simulink model "FullSystemSimFinal_sexy"  (R2020a)
settings: Solver=ode23t  StartTime=0.0  StopTime=T_sim  MaxStep=0.0005  RelTol=1e-3
values from neighbouring files (symbols this model uses):
  a_friction = 0    [FullSystem.m]
  b_friction = 1.19    [FullSystem.m]
  C_T_matrix = ex2(2:12,2:12)'    [FullSystem.m]
  d_turbine = 0.15    [FullSystem.m]
  I_mp_data = ex4(:,5)    [FullSystem.m]
  I_sc_data = ex4(:,3)    [FullSystem.m]
  J_wind = 5.245e-6 * 1000    (= 0.005245)    [FullSystem.m]
  K_t = 0.023    [FullSystem.m]    (also in WindTurbine.m = 82.8991502528)
  K_v = 0.023 * pi / 30    (= 0.00240855436775)    [FullSystem.m]    (also in WindTurbine.m = 115.191730632)
  lambda_data_x = ex3(3, :)'    [FullSystem.m]
  lambda_opt = 2.8    [FullSystem.m]
  omega_0 = 1000    [FullSystem.m]    (also in SystemControl_script.m = 100:)
  P_max_EL = 3    [FullSystem.m]
  P_max_FC = 1    [FullSystem.m]
  R_LED_max = 75/4    (= 18.75)    [FullSystem.m]
  r_LED_x = ex1(4, :)'    [FullSystem.m]
  R_mp_data = ex4(:,6)    [FullSystem.m]
  r_PS_x = ex1(5,:)'    [FullSystem.m]
  r_solar_data_x = ex4(:,1)    [FullSystem.m]
  r_SP_x = ex1(3, :)'    [FullSystem.m]
  r_wind_data_x = ex3(1, :)'    [FullSystem.m]
  r_WT_x = ex1(2, :)'    [FullSystem.m]
  rho_air = 1.225    [FullSystem.m]
  step_size = T_sim/n    (= 0.01)    [FullSystem.m]
  T_sim = 10    [FullSystem.m]    (also in SystemControl_script.m; model_1.m = 24)
  V_mp_data = ex4(:,4)    [FullSystem.m]
  V_oc_data = ex4(:,2)    [FullSystem.m]
  V_w_data_x = ex3(2,:)'    [FullSystem.m]
undefined symbols (not defined in the file or in its folder): DiscIntNeverNeededParam
libraries: fl_lib x54, nesl_utility x49, simulink x2, ee_lib x1
settings Model: Creator=thequ  LastModifiedBy=thequ
settings DebuggingCC: SignalInfNanChecking=warning  ArithmeticOperatorsInVariantConditions=warning
settings SFSimCC: CustomCodeUndefinedFunction=UseInterfaceOnly

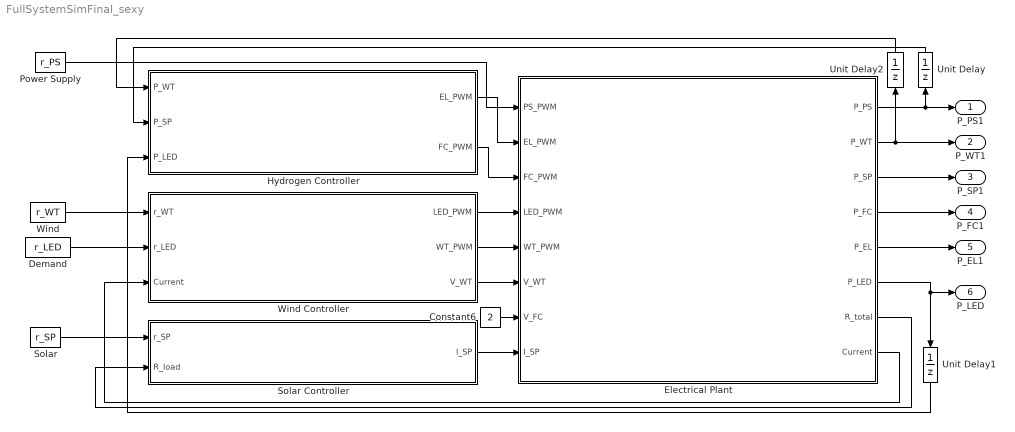
== system FullSystemSimFinal_sexy ==
  Constant6 : Constant  Value=2
  Demand : FromWorkspace  VariableName=r_LED  SampleTime=T_sim/length(r_LED_x)  Interpolate=off  OutputAfterFinalValue=Holding final value
  Electrical Plant : Subsystem
  Hydrogen Controller : Subsystem
  Power Supply : FromWorkspace  VariableName=r_PS  SampleTime=T_sim/length(r_PS_x)  Interpolate=off  OutputAfterFinalValue=Holding final value
  Solar : FromWorkspace  VariableName=r_SP  SampleTime=T_sim/length(r_SP_x)  Interpolate=off  OutputAfterFinalValue=Holding final value
  Solar Controller : Subsystem
  Unit Delay : UnitDelay  SampleTime=-1  HasFrameUpgradeWarning=on
  Unit Delay1 : UnitDelay  SampleTime=-1  HasFrameUpgradeWarning=on
  Unit Delay2 : UnitDelay  SampleTime=-1  HasFrameUpgradeWarning=on
  Wind : FromWorkspace  VariableName=r_WT  SampleTime=T_sim/length(r_WT_x)  Interpolate=off  OutputAfterFinalValue=Holding final value
  Wind Controller : Subsystem
  P_PS1 : Outport
  P_WT1 : Outport  Port=2
  P_SP1 : Outport  Port=3
  P_FC1 : Outport  Port=4
  P_EL1 : Outport  Port=5
  P_LED : Outport  Port=6
  wires:
  Electrical Plant/1(P_PS) -> P_PS1/1, Unit Delay/1
  Electrical Plant/2(P_WT) -> P_WT1/1, Unit Delay2/1
  Electrical Plant/3(P_SP) -> P_SP1/1
  Electrical Plant/4(P_FC) -> P_FC1/1
  Electrical Plant/5(P_EL) -> P_EL1/1
  Demand/1 -> Wind Controller/2(r_LED)
  Constant6/1 -> Electrical Plant/7(V_FC)
  Wind/1 -> Wind Controller/1(r_WT)
  Wind Controller/2(WT_PWM) -> Electrical Plant/5(WT_PWM)
  Power Supply/1 -> Electrical Plant/1(PS_PWM)
  Hydrogen Controller/1(EL_PWM) -> Electrical Plant/2(EL_PWM)
  Hydrogen Controller/2(FC_PWM) -> Electrical Plant/3(FC_PWM)
  Wind Controller/1(LED_PWM) -> Electrical Plant/4(LED_PWM)
  Wind Controller/3(V_WT) -> Electrical Plant/6(V_WT)
  Electrical Plant/8(Current) -> Wind Controller/3(Current)
  Electrical Plant/6(P_LED) -> P_LED/1, Unit Delay1/1
  Unit Delay/1 -> Hydrogen Controller/2(P_SP)
  Unit Delay1/1 -> Hydrogen Controller/3(P_LED)
  Unit Delay2/1 -> Hydrogen Controller/1(P_WT)
  Solar Controller/1(I_SP) -> Electrical Plant/8(I_SP)
  Solar/1 -> Solar Controller/1(r_SP)
  Electrical Plant/7(R_total) -> Solar Controller/2(R_load)

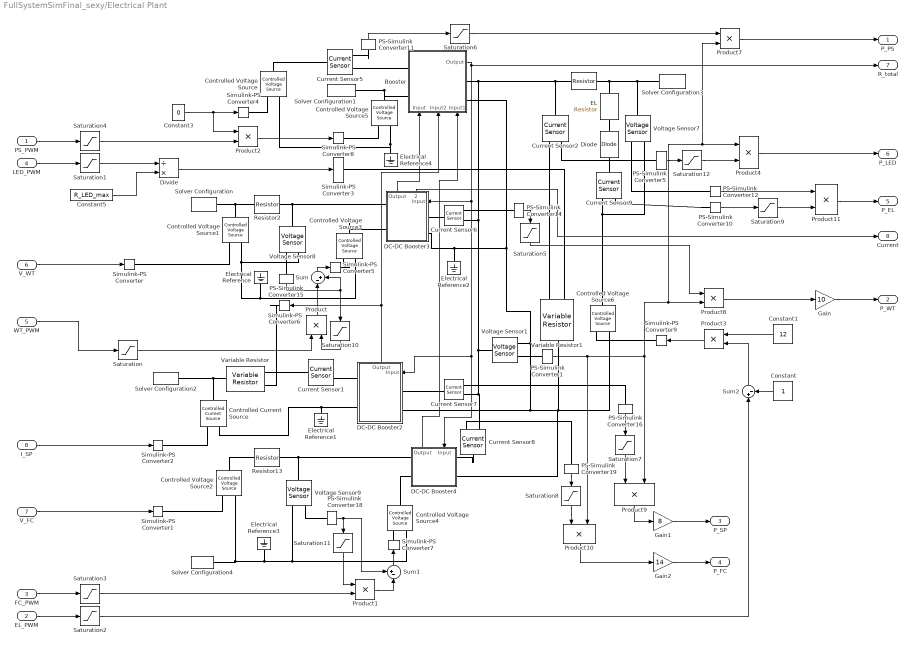
== system FullSystemSimFinal_sexy/Electrical Plant ==
  PS_PWM : Inport
  EL_PWM : Inport  Port=2
  FC_PWM : Inport  Port=3
  LED_PWM : Inport  Port=4
  WT_PWM : Inport  Port=5
  V_WT : Inport  Port=6
  V_FC : Inport  Port=7
  I_SP : Inport  Port=8
  " " : fl_lib/Electrical/Electrical Elements/Resistor  R=16 Ohm  i_specify=off  i_priority=None  i=0 A  i_nominal_specify=off  i_nominal_unit=A  i_nominal_value=1  v_specify=off  v_priority=None  v=0 V  v_nominal_specify=off  v_nominal_unit=V  v_nominal_value=1
  Booster : Subsystem
      settings: PortSchema="{\"entries\":[{\"content\":{\"sides\":[{\"content\":{\"connectorIds\":[\"LConn1\",\"LConn2\"]},\"type\":\"ConnectorPlacement.EquallySpacedRectSide\",\"uuid\":\"3f87025d-e72c-4f7c-9c78-5492fcc5bb7b\"},{\"content\":{\"connectorIds\":[\"Out1\",\"RConn1\",\"RConn2\"],\"side\":\"RIGHT\"},\"type\":\"ConnectorPlacement.EquallySpacedRectSide\",\"uuid\":\"8496db32-d1b8-4ca7-babe-2510a055e486\"},{\"content\":{\"connectorIds\":[],\"side\":\"TOP\"},\"type\":\"ConnectorPlacement.EquallySpacedRectSide\",\"uuid\":\"d85b2c98-f560-4129-a6ac-6fa684551bcf\"},{\"content\":{\"connectorIds\":[\"In1\",\"In2\",\"In3\"],\"side\":\"BOTTOM\"},\"type\":\"ConnectorPlacement.EquallySpacedRectSide\",\"uuid\":\"fe0eaf9c-8c75-4de4-84e6-0314a1617f55\"}]},\"type\":\"ConnectorPlacement.EquallySpacedConnector\",\"uuid\":\"a6ed506c-6875-4055-9614-7dad2b572790\"}],\"packageUris\":[\"http://schema.mathworks.com/mf0/Connector/19700101\"],\"version\":\"1.0\"}"
  Constant : Constant
  Constant1 : Constant  Value=12
  Constant3 : Constant  Value=0
  Constant5 : Constant  Value=R_LED_max
  Controlled Current Source : fl_lib/Electrical/Electrical Sources/Controlled Current Source
  Controlled Voltage Source{,1..6} (7 alike) : fl_lib/Electrical/Electrical Sources/Controlled Voltage Source
  Current Sensor{1..2,5..9} (7 alike) : fl_lib/Electrical/Electrical Sensors/Current Sensor
  DC-DC Booster2 : Subsystem
      settings: PortSchema="{\"entries\":[{\"content\":{\"sides\":[{\"content\":{\"connectorIds\":[\"LConn1\",\"LConn2\"]},\"type\":\"ConnectorPlacement.EquallySpacedRectSide\",\"uuid\":\"e779e15f-05fe-47ae-aa08-5379ba170b98\"},{\"content\":{\"connectorIds\":[\"In1\",\"RConn1\",\"RConn2\"],\"side\":\"RIGHT\"},\"type\":\"ConnectorPlacement.EquallySpacedRectSide\",\"uuid\":\"c806a98b-8847-4c98-ba30-df3a6a47e20e\"},{\"content\":{\"connectorIds\":[\"Out1\"],\"side\":\"TOP\"},\"type\":\"ConnectorPlacement.EquallySpacedRectSide\",\"uuid\":\"f525c8fa-41c3-4ddc-a882-4dcfcc470e8d\"}]},\"type\":\"ConnectorPlacement.EquallySpacedConnector\",\"uuid\":\"8e1dab04-976c-405f-8e86-df668b770438\"}],\"packageUris\":[\"http://schema.mathworks.com/mf0/Connector/19700101\"],\"version\":\"1.0\"}"
  DC-DC Booster3 : Subsystem
      settings: PortSchema="{\"entries\":[{\"content\":{\"sides\":[{\"content\":{\"connectorIds\":[\"LConn1\",\"LConn2\"]},\"type\":\"ConnectorPlacement.EquallySpacedRectSide\",\"uuid\":\"e779e15f-05fe-47ae-aa08-5379ba170b98\"},{\"content\":{\"connectorIds\":[\"In1\",\"RConn1\",\"RConn2\"],\"side\":\"RIGHT\"},\"type\":\"ConnectorPlacement.EquallySpacedRectSide\",\"uuid\":\"c806a98b-8847-4c98-ba30-df3a6a47e20e\"},{\"content\":{\"connectorIds\":[\"Out1\",\"Out2\"],\"side\":\"TOP\"},\"type\":\"ConnectorPlacement.EquallySpacedRectSide\",\"uuid\":\"f525c8fa-41c3-4ddc-a882-4dcfcc470e8d\"}]},\"type\":\"ConnectorPlacement.EquallySpacedConnector\",\"uuid\":\"8e1dab04-976c-405f-8e86-df668b770438\"}],\"packageUris\":[\"http://schema.mathworks.com/mf0/Connector/19700101\"],\"version\":\"1.0\"}"
  DC-DC Booster4 : Subsystem
      settings: PortSchema="{\"entries\":[{\"content\":{\"sides\":[{\"content\":{\"connectorIds\":[\"LConn1\",\"LConn2\"]},\"type\":\"ConnectorPlacement.EquallySpacedRectSide\",\"uuid\":\"53e27ef1-b6e4-4838-a313-2833a9f48f28\"},{\"content\":{\"connectorIds\":[\"RConn1\",\"RConn2\"],\"side\":\"RIGHT\"},\"type\":\"ConnectorPlacement.EquallySpacedRectSide\",\"uuid\":\"d6eb4206-926e-4a9e-8f3b-898e00b2f09a\"},{\"content\":{\"connectorIds\":[\"Out1\",\"In1\"],\"side\":\"TOP\"},\"type\":\"ConnectorPlacement.EquallySpacedRectSide\",\"uuid\":\"2a6192b7-9850-4397-b133-a2a3e44eb736\"}]},\"type\":\"ConnectorPlacement.EquallySpacedConnector\",\"uuid\":\"90d1bf23-e581-4b0f-8608-623e9f776cda\"}],\"packageUris\":[\"http://schema.mathworks.com/mf0/Connector/19700101\"],\"version\":\"1.0\"}"
  Diode : ee_lib/Semiconductors & Converters/Diode  ModelType=ee.enum.diode.modelType.pwl  Vf=0.6 V  Ron=0.3 Ohm  Goff=1e-8 S  prmExp=ee.enum.diode.expParam.useTwo  I12=[.0137, .545] A  V12=[.6, .7] V  IS=1e-12 A  ec=1  I1=0.0137 A  V1=0.6 V  RS=0 Ohm  Tmeas=25 degC  N_series=1  N_parallel=1  Rz=0.2 Ohm  BV=1.51 V  C_param=ee.enum.diode.capParam.fixed  CJ=5 pF  CJ0=5 pF  VJ=1 V  Mgrad=0.5  Vvec=[.1, 10, 100] V  Cvec=[3.5, 1, .4] pF  FC=0.5  Q_param=ee.enum.diode.recoveryParam.off  iRM=-7.15 A  iF=4 A  didt=-750 A/us  trr_factor=3  trr=115 ns  Qrr=1500 s*uA  TT=50 ns  tau=100 ns  T_param=ee.enum.diode.temperatureParam.off  IS_T2=1.25e-7 A  I1_T2=0.245 A  V1_T2=0.5 V  Tmeas2=125 degC  EG_param=ee.enum.diode.egapParam.material_si  EG=1.11 eV  XTI_param=ee.enum.diode.xtiParam.pn  XTI=3  dBVdT=0 V/K  Tdevice=25 degC  i_specify=off  i_priority=None  i=0 A  i_nominal_specify=off  i_nominal_unit=A  i_nominal_value=1  v_specify=off  v_priority=None  v=0 V  v_nominal_specify=off  v_nominal_unit=V  v_nominal_value=1  i_capacitor_specify=off  i_capacitor_priority=None  i_capacitor=0 A  i_capacitor_nominal_specify=off  i_capacitor_nominal_unit=A  i_capacitor_nominal_value=1  v_capacitor_specify=off  v_capacitor_priority=None  v_capacitor=0 V  v_capacitor_nominal_specify=off  v_capacitor_nominal_unit=V  v_capacitor_nominal_value=1  power_dissipated_specify=off  power_dissipated_priority=None  power_dissipated=0 W  power_dissipated_nominal_specify=off  power_dissipated_nominal_unit=W  power_dissipated_nominal_value=1  thermal_network_parameterization=ee.enum.thermalNetworkTopology.cauer  Rth=[0, 10] K/W  Rth_Foster=[4, 6] K/W  thermal_mass_parameterization=ee.enum.thermalNetwork.timeconstant  thermal_mass=[0, 1] J/K  thermal_mass_Foster=[1.5, 3] J/K  thermal_time_constant=[0, 10] s  thermal_time_constant_Foster=[6, 18] s  thermal_mass_initial_temperatures=[25, 25] degC
  Divide : Product  Inputs=/*
  EL : fl_lib/Electrical/Electrical Elements/Resistor  R=3 Ohm  i_specify=off  i_priority=None  i=0 A  i_nominal_specify=off  i_nominal_unit=A  i_nominal_value=1  v_specify=off  v_priority=None  v=0 V  v_nominal_specify=off  v_nominal_unit=V  v_nominal_value=1
  Electrical Reference{,1..4} (5 alike) : fl_lib/Electrical/Electrical Elements/Electrical Reference
  Gain : Gain  Gain=10
  Gain1 : Gain  Gain=8
  Gain2 : Gain  Gain=14
  PS-Simulink Converter{1,5,10..12,14,16,18..19} (9 alike) : nesl_utility/PS-Simulink Converter  PhysicalDomain=network_engine_domain  SubClassName=ps_output  LeftPortType=input  RightPortType=output  PseudoPeriodic=off  Frequencies=[]  Unit=inherit  AffineConversion=off
  PS-Simulink Converter15 : nesl_utility/PS-Simulink Converter  PhysicalDomain=network_engine_domain  SubClassName=ps_output  LeftPortType=input  RightPortType=output  PseudoPeriodic=off  Frequencies=[]  Unit=inherit  AffineConversion=on
  Product{,1..4,7..11} (10 alike) : Product
  Resistor13 : fl_lib/Electrical/Electrical Elements/Resistor  R=16 Ohm  i_specify=off  i_priority=None  i=0 A  i_nominal_specify=off  i_nominal_unit=A  i_nominal_value=1  v_specify=off  v_priority=None  v=0 V  v_nominal_specify=off  v_nominal_unit=V  v_nominal_value=1
  Resistor2 : fl_lib/Electrical/Electrical Elements/Resistor  R=16 Ohm  i_specify=off  i_priority=None  i=0 A  i_nominal_specify=off  i_nominal_unit=A  i_nominal_value=1  v_specify=off  v_priority=None  v=0 V  v_nominal_specify=off  v_nominal_unit=V  v_nominal_value=1
  Saturation : Saturate  UpperLimit=1  LowerLimit=0.01
  Saturation1 : Saturate  UpperLimit=1  LowerLimit=0.01
  Saturation10 : Saturate  UpperLimit=12  LowerLimit=0.01
  Saturation11 : Saturate  UpperLimit=12  LowerLimit=0.01
  Saturation12 : Saturate  UpperLimit=2  LowerLimit=0
  Saturation{2..4,7} (4 alike) : Saturate  UpperLimit=1  LowerLimit=0
  Saturation5 : Saturate  UpperLimit=2
  Saturation6 : Saturate  UpperLimit=2
  Saturation8 : Saturate
  Saturation9 : Saturate  UpperLimit=2  LowerLimit=0  ZeroCross=off
  Simulink-PS Converter{,2..3,5..9} (8 alike) : nesl_utility/Simulink-PS Converter  PhysicalDomain=network_engine_domain  SubClassName=ps_input  LeftPortType=input  RightPortType=output  PseudoPeriodic=off  Frequencies=[]  NoiseDistribution=none  NoiseParameters=[]  Unit=1  AffineConversion=off  FilteringAndDerivatives=filter  SimscapeFilterOrder=1  InputFilterTimeConstant=0.001  UdotUserProvided=0
  Simulink-PS Converter1 : nesl_utility/Simulink-PS Converter  PhysicalDomain=network_engine_domain  SubClassName=ps_input  LeftPortType=input  RightPortType=output  PseudoPeriodic=off  Frequencies=[]  NoiseDistribution=none  NoiseParameters=[]  Unit=1  AffineConversion=off  FilteringAndDerivatives=provide  SimscapeFilterOrder=1  InputFilterTimeConstant=0.001  UdotUserProvided=0
  Simulink-PS Converter4 : nesl_utility/Simulink-PS Converter  PhysicalDomain=network_engine_domain  SubClassName=ps_input  LeftPortType=input  RightPortType=output  PseudoPeriodic=off  Frequencies=[]  NoiseDistribution=none  NoiseParameters=[]  Unit=1  AffineConversion=off  FilteringAndDerivatives=provide  SimscapeFilterOrder=1  InputFilterTimeConstant=0.001  UdotUserProvided=0
  Solver Configuration : nesl_utility/Solver Configuration  PhysicalDomain=network_engine_domain  SubClassName=solver  LeftPortType=input  RightPortType=generic  Tones=[]  Harmonics=[]  SimulateNoise=off  Profile=off  UseLocalSampling=off  EnableSwitchedLinearOptims=on  FrequencyDomain=off  UseCCode=off  RelTol=0.001  AbsTol=1e-06  MinStep=1e-09  ToWorkspace=off  RevertToSquareIcSolve=off  NumHomotopyIterations=100  PhasorMode=off  PhasorModeNumHarmonics=1  DoDC=on  ResidualTolerance=1e-09  UseLocalSolver=off  LocalSolverChoice=NE_TRAPEZOIDAL_ADVANCER  LocalSolverSampleTime=0.001  DoFixedCost=off  MaxNonlinIter=3  MaxModeIter=2  LinearAlgebra=auto  EquationFormulation=NE_TIME_EF  DelaysMemoryBudget=1024  AutomaticFiltering=on  FilteringTimeConstant=0.001  PartitionStorageMethod=AS_NEEDED  PartitionMemoryBudget=1024  PartitionMethod=ROBUST
  Solver Configuration1 : nesl_utility/Solver Configuration  PhysicalDomain=network_engine_domain  SubClassName=solver  LeftPortType=input  RightPortType=generic  Tones=[]  Harmonics=[]  SimulateNoise=off  Profile=off  UseLocalSampling=off  EnableSwitchedLinearOptims=on  FrequencyDomain=off  UseCCode=off  RelTol=0.001  AbsTol=1e-06  MinStep=1e-09  ToWorkspace=off  RevertToSquareIcSolve=off  NumHomotopyIterations=100  PhasorMode=off  PhasorModeNumHarmonics=1  DoDC=on  ResidualTolerance=1e-9  UseLocalSolver=off  LocalSolverChoice=NE_BACKWARD_EULER_ADVANCER  LocalSolverSampleTime=0.001  DoFixedCost=off  MaxNonlinIter=3  MaxModeIter=2  LinearAlgebra=auto  EquationFormulation=NE_TIME_EF  DelaysMemoryBudget=1024  AutomaticFiltering=on  FilteringTimeConstant=0.001  PartitionStorageMethod=AS_NEEDED  PartitionMemoryBudget=1024  PartitionMethod=ROBUST
  Solver Configuration2 : nesl_utility/Solver Configuration  PhysicalDomain=network_engine_domain  SubClassName=solver  LeftPortType=input  RightPortType=generic  Tones=[]  Harmonics=[]  SimulateNoise=off  Profile=off  UseLocalSampling=off  EnableSwitchedLinearOptims=on  FrequencyDomain=off  UseCCode=off  RelTol=0.001  AbsTol=1e-06  MinStep=1e-09  ToWorkspace=off  RevertToSquareIcSolve=off  NumHomotopyIterations=100  PhasorMode=off  PhasorModeNumHarmonics=1  DoDC=on  ResidualTolerance=1e-3  UseLocalSolver=off  LocalSolverChoice=NE_BACKWARD_EULER_ADVANCER  LocalSolverSampleTime=0.001  DoFixedCost=off  MaxNonlinIter=3  MaxModeIter=2  LinearAlgebra=auto  EquationFormulation=NE_TIME_EF  DelaysMemoryBudget=1024  AutomaticFiltering=on  FilteringTimeConstant=0.001  PartitionStorageMethod=AS_NEEDED  PartitionMemoryBudget=1024  PartitionMethod=ROBUST
  Solver Configuration3 : nesl_utility/Solver Configuration  PhysicalDomain=network_engine_domain  SubClassName=solver  LeftPortType=input  RightPortType=generic  Tones=[]  Harmonics=[]  SimulateNoise=off  Profile=off  UseLocalSampling=off  EnableSwitchedLinearOptims=on  FrequencyDomain=off  UseCCode=off  RelTol=0.001  AbsTol=1e-06  MinStep=1e-09  ToWorkspace=off  RevertToSquareIcSolve=off  NumHomotopyIterations=100  PhasorMode=off  PhasorModeNumHarmonics=1  DoDC=on  ResidualTolerance=1e-6  UseLocalSolver=off  LocalSolverChoice=NE_BACKWARD_EULER_ADVANCER  LocalSolverSampleTime=0.001  DoFixedCost=off  MaxNonlinIter=3  MaxModeIter=2  LinearAlgebra=Full  EquationFormulation=NE_TIME_EF  DelaysMemoryBudget=2048  AutomaticFiltering=on  FilteringTimeConstant=0.001  PartitionStorageMethod=AS_NEEDED  PartitionMemoryBudget=1024  PartitionMethod=ROBUST
  Solver Configuration4 : nesl_utility/Solver Configuration  PhysicalDomain=network_engine_domain  SubClassName=solver  LeftPortType=input  RightPortType=generic  Tones=[]  Harmonics=[]  SimulateNoise=off  Profile=off  UseLocalSampling=off  EnableSwitchedLinearOptims=on  FrequencyDomain=off  UseCCode=off  RelTol=0.001  AbsTol=1e-06  MinStep=1e-09  ToWorkspace=off  RevertToSquareIcSolve=off  NumHomotopyIterations=100  PhasorMode=off  PhasorModeNumHarmonics=1  DoDC=on  ResidualTolerance=1e-9  UseLocalSolver=off  LocalSolverChoice=NE_BACKWARD_EULER_ADVANCER  LocalSolverSampleTime=0.001  DoFixedCost=off  MaxNonlinIter=3  MaxModeIter=2  LinearAlgebra=auto  EquationFormulation=NE_TIME_EF  DelaysMemoryBudget=1024  AutomaticFiltering=on  FilteringTimeConstant=0.001  PartitionStorageMethod=AS_NEEDED  PartitionMemoryBudget=1024  PartitionMethod=ROBUST
  Sum : Sum  Inputs=|-+
  Sum1 : Sum  Inputs=+-|
  Sum2 : Sum  Inputs=|+-
  Variable Resistor : fl_lib/Electrical/Electrical Elements/Variable Resistor  Rmin=0 Ohm  i_specify=off  i_priority=None  i=0 A  i_nominal_specify=off  i_nominal_unit=A  i_nominal_value=1  v_specify=off  v_priority=None  v=0 V  v_nominal_specify=off  v_nominal_unit=V  v_nominal_value=1
  Variable Resistor1 : fl_lib/Electrical/Electrical Elements/Variable Resistor  Rmin=1 Ohm  i_specify=off  i_priority=None  i=0 A  i_nominal_specify=off  i_nominal_unit=A  i_nominal_value=1  v_specify=off  v_priority=None  v=0 V  v_nominal_specify=off  v_nominal_unit=V  v_nominal_value=1
  Voltage Sensor{1,7..9} (4 alike) : fl_lib/Electrical/Electrical Sensors/Voltage Sensor
  P_PS : Outport
  P_WT : Outport  Port=2
  P_SP : Outport  Port=3
  P_FC : Outport  Port=4
  P_EL : Outport  Port=5
  P_LED : Outport  Port=6
  R_total : Outport  Port=7
  Current : Outport  Port=8
  wires:
  PS_PWM/1 -> Saturation4/1
  WT_PWM/1 -> Saturation/1
  Divide/1 -> Simulink-PS Converter3/1
  PS-Simulink Converter11/1 -> Saturation6/1
  Product11/1 -> P_EL/1
  FC_PWM/1 -> Saturation3/1
  EL_PWM/1 -> Saturation2/1
  Product9/1 -> Gain1/1
  Constant5/1 -> Divide/2
  PS-Simulink Converter18/1 -> Saturation11/1, Sum1/1
  PS-Simulink Converter10/1 -> Saturation9/1
  V_WT/1 -> Simulink-PS Converter/1
  Product8/1 -> Gain/1
  Product10/1 -> Gain2/1
  V_FC/1 -> Simulink-PS Converter1/1
  Product7/1 -> P_PS/1
  LED_PWM/1 -> Saturation1/1
  PS-Simulink Converter12/1 -> Product11/1
  PS-Simulink Converter19/1 -> Saturation8/1
  PS-Simulink Converter14/1 -> Saturation5/1
  PS-Simulink Converter15/1 -> Saturation10/1, Sum/2
  Constant3/1 -> Product2/1, Simulink-PS Converter4/1
  Saturation1/1 -> Divide/1
  Saturation2/1 -> Sum2/1
  Saturation3/1 -> Product1/2
  Saturation4/1 -> Product2/2
  Saturation/1 -> Product/1
  I_SP/1 -> Simulink-PS Converter2/1
  PS-Simulink Converter16/1 -> Saturation7/1
  Saturation5/1 -> Product8/1
  Saturation6/1 -> Product7/1
  Saturation7/1 -> Product9/1
  Saturation8/1 -> Product10/1
  Saturation9/1 -> Product11/2
  Booster/1(Output) -> DC-DC Booster3/1(Input), DC-DC Booster4/1(Input), DC-DC Booster2/1(Input), R_total/1
  DC-DC Booster3/1(Output) -> Booster/1(Input)
  DC-DC Booster2/1(Output) -> Simulink-PS Converter6/1, Booster/2(Input2)
  DC-DC Booster4/1(Output) -> Booster/3(Input1)
  DC-DC Booster3/2(Output1) -> Current/1
  Sum/1 -> Simulink-PS Converter5/1
  Product/1 -> Sum/1
  Saturation10/1 -> Product/2
  Sum1/1 -> Simulink-PS Converter7/1
  Saturation11/1 -> Product1/1
  Product1/1 -> Sum1/2
  Product2/1 -> Simulink-PS Converter8/1
  Constant1/1 -> Product3/1
  Product3/1 -> Simulink-PS Converter9/1
  Product4/1 -> P_LED/1
  Saturation12/1 -> Product4/2
  PS-Simulink Converter1/1 -> Product8/2, Product7/2, Product4/1, Product9/2, Product10/2
  Sum2/1 -> Product3/2
  Constant/1 -> Sum2/2
  PS-Simulink Converter5/1 -> Saturation12/1
  Gain/1 -> P_WT/1
  Gain1/1 -> P_SP/1
  Gain2/1 -> P_FC/1
  connections:
  Simulink-PS Converter4/RConn1 -- Controlled Voltage Source/RConn1
  Current Sensor9/RConn2 -- Voltage Sensor7/RConn2 -- Controlled Voltage Source6/LConn1
  Booster/LConn2 -- Controlled Voltage Source5/LConn1 -- Solver Configuration1/RConn1
  Voltage Sensor9/LConn1 -- DC-DC Booster4/LConn1 -- Resistor13/RConn1
  " "/RConn1 -- Voltage Sensor7/LConn1 -- Solver Configuration3/RConn1 -- EL/LConn1
  DC-DC Booster2/LConn1 -- Current Sensor1/RConn2
  DC-DC Booster4/LConn2 -- Controlled Voltage Source4/LConn1
  Resistor13/LConn1 -- Controlled Voltage Source2/LConn1
  Simulink-PS Converter3/RConn1 -- Variable Resistor1/LConn1
  PS-Simulink Converter11/LConn1 -- Current Sensor5/RConn1
  Simulink-PS Converter1/RConn1 -- Controlled Voltage Source2/RConn1
  Simulink-PS Converter/RConn1 -- Controlled Voltage Source1/RConn1
  PS-Simulink Converter18/LConn1 -- Voltage Sensor9/RConn1
  Current Sensor6/RConn1 -- PS-Simulink Converter14/LConn1
  PS-Simulink Converter15/LConn1 -- Voltage Sensor8/RConn1
  Current Sensor7/RConn1 -- PS-Simulink Converter16/LConn1
  PS-Simulink Converter19/LConn1 -- Current Sensor8/RConn1
  Controlled Voltage Source/LConn1 -- Current Sensor5/LConn1
  PS-Simulink Converter12/LConn1 -- Voltage Sensor7/RConn1
  Simulink-PS Converter2/RConn1 -- Controlled Current Source/RConn1
  PS-Simulink Converter10/LConn1 -- Current Sensor9/RConn1
  PS-Simulink Converter1/LConn1 -- Voltage Sensor1/RConn1
  Current Sensor6/LConn1 -- DC-DC Booster3/RConn1
  DC-DC Booster4/RConn1 -- Current Sensor8/LConn1
  Current Sensor7/LConn1 -- DC-DC Booster2/RConn1
  Controlled Current Source/RConn2 -- DC-DC Booster2/LConn2 -- Electrical Reference1/LConn1
  Variable Resistor/LConn2 -- Current Sensor1/LConn1
  DC-DC Booster3/LConn1 -- Resistor2/RConn1 -- Voltage Sensor8/LConn1
  Controlled Voltage Source5/RConn2 -- Electrical Reference4/LConn1 -- Controlled Voltage Source/RConn2
  Controlled Voltage Source2/RConn2 -- Voltage Sensor9/RConn2 -- Controlled Voltage Source4/RConn2 -- Electrical Reference3/LConn1 -- Solver Configuration4/RConn1
  Current Sensor5/RConn2 -- Booster/LConn1
  Controlled Voltage Source1/LConn1 -- Solver Configuration/RConn1 -- Resistor2/LConn1
  " "/LConn1 -- Voltage Sensor1/LConn1 -- Current Sensor8/RConn2 -- Current Sensor7/RConn2 -- Current Sensor6/RConn2 -- Booster/RConn1 -- Current Sensor2/LConn1
  Voltage Sensor8/RConn2 -- Controlled Voltage Source1/RConn2 -- Controlled Voltage Source3/RConn2 -- Electrical Reference/LConn1
  Controlled Voltage Source3/LConn1 -- DC-DC Booster3/LConn2
  Simulink-PS Converter5/RConn1 -- Controlled Voltage Source3/RConn1
  Simulink-PS Converter7/RConn1 -- Controlled Voltage Source4/RConn1
  Simulink-PS Converter8/RConn1 -- Controlled Voltage Source5/RConn1
  Variable Resistor1/RConn1 -- Controlled Voltage Source6/RConn2 -- Booster/RConn2 -- DC-DC Booster3/RConn2 -- Electrical Reference2/LConn1 -- Voltage Sensor1/RConn2 -- DC-DC Booster2/RConn2 -- DC-DC Booster4/RConn2
  Controlled Voltage Source6/RConn1 -- Simulink-PS Converter9/RConn1
  Variable Resistor1/LConn2 -- Current Sensor2/RConn2
  Current Sensor2/RConn1 -- PS-Simulink Converter5/LConn1
  Solver Configuration2/RConn1 -- Variable Resistor/RConn1 -- Controlled Current Source/LConn1
  Simulink-PS Converter6/RConn1 -- Variable Resistor/LConn1
  Diode/RConn1 -- EL/RConn1
  Diode/LConn1 -- Current Sensor9/LConn1

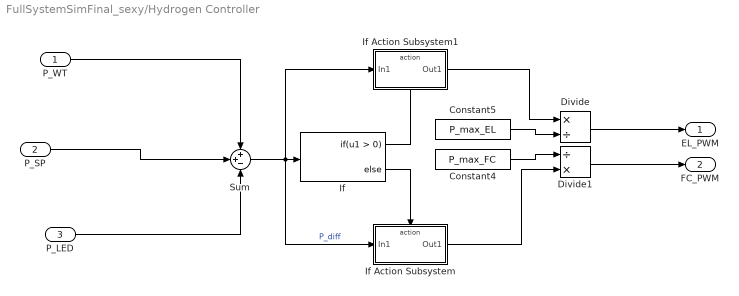
== system FullSystemSimFinal_sexy/Hydrogen Controller ==
  P_WT : Inport
  P_SP : Inport  Port=2
  P_LED : Inport  Port=3
  Constant4 : Constant  Value=P_max_FC
  Constant5 : Constant  Value=P_max_EL
  Divide : Product  Inputs=*/
  Divide1 : Product  Inputs=/*
  If : If
  If Action Subsystem : Subsystem  TreatAsAtomicUnit=on
  If Action Subsystem1 : Subsystem  TreatAsAtomicUnit=on
  Sum : Sum  Inputs=++-
  EL_PWM : Outport
  FC_PWM : Outport  Port=2
  wires:
  Divide1/1 -> FC_PWM/1
  Divide/1 -> EL_PWM/1
  If Action Subsystem/1(Out1) -> Divide1/2
  Constant5/1 -> Divide/2
  If/2 -> If Action Subsystem/Action
  Sum/1 -> If Action Subsystem1/1(In1), If Action Subsystem/1(In1), If/1  "P_diff"
  Constant4/1 -> Divide1/1
  If/1 -> If Action Subsystem1/Action
  If Action Subsystem1/1(Out1) -> Divide/1
  P_WT/1 -> Sum/1
  P_SP/1 -> Sum/2
  P_LED/1 -> Sum/3

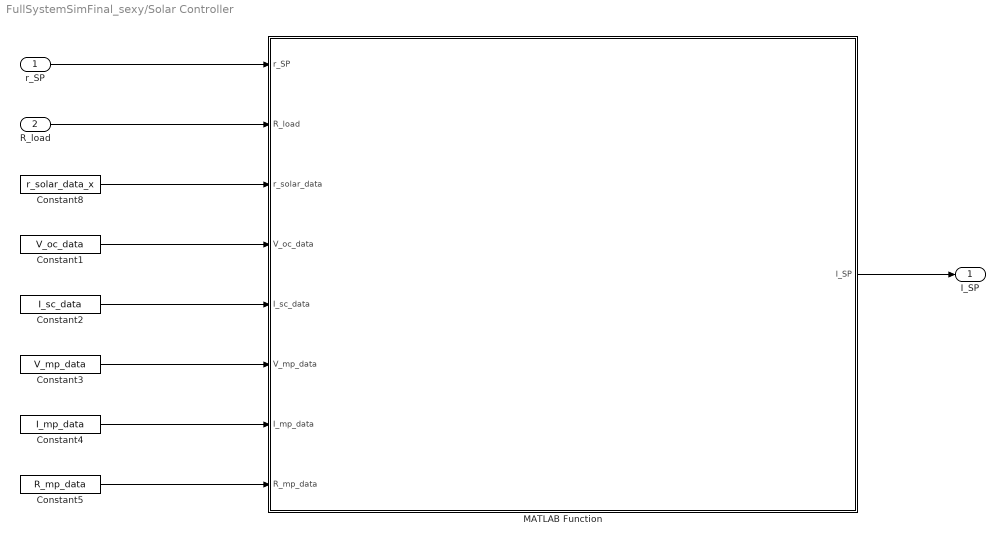
== system FullSystemSimFinal_sexy/Solar Controller ==
  r_SP : Inport
  R_load : Inport  Port=2
  Constant1 : Constant  Value=V_oc_data
  Constant2 : Constant  Value=I_sc_data
  Constant3 : Constant  Value=V_mp_data
  Constant4 : Constant  Value=I_mp_data
  Constant5 : Constant  Value=R_mp_data
  Constant8 : Constant  Value=r_solar_data_x
  MATLAB Function : MATLAB Function  TreatAsAtomicUnit=on
  I_SP : Outport
  wires:
  r_SP/1 -> MATLAB Function/1(r_SP)
  Constant8/1 -> MATLAB Function/3(r_solar_data)
  R_load/1 -> MATLAB Function/2(R_load)
  MATLAB Function/1(I_SP) -> I_SP/1
  Constant1/1 -> MATLAB Function/4(V_oc_data)
  Constant4/1 -> MATLAB Function/7(I_mp_data)
  Constant5/1 -> MATLAB Function/8(R_mp_data)
  Constant3/1 -> MATLAB Function/6(V_mp_data)
  Constant2/1 -> MATLAB Function/5(I_sc_data)

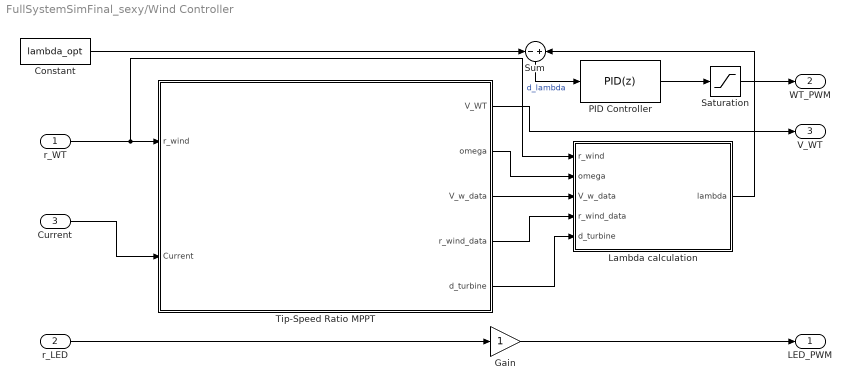
== system FullSystemSimFinal_sexy/Wind Controller ==
  r_WT : Inport
  r_LED : Inport  Port=2
  Current : Inport  Port=3
  Constant : Constant  Value=lambda_opt
  Gain : Gain
  Lambda calculation : Subsystem
  PID Controller : simulink/Continuous/PID Controller  Controller=PID  Form=Parallel  TimeDomain=Discrete-time  UseExternalTs=off  SampleTime=-1  IntegratorMethod=Forward Euler  FilterMethod=Forward Euler  ControllerParametersSource=internal  P=10  I=0.1  D=0  UseFilter=on  N=100  TunerSelectOption=Transfer Function Based (PID Tuner App)  InitialConditionSource=internal  InitialConditionForIntegrator=0  InitialConditionForFilter=0  DifferentiatorICPrevScaledInput=0  ExternalReset=none  TrackingMode=off  Kt=1  LimitOutput=off  UpperSaturationLimit=inf  LowerSaturationLimit=-inf  LinearizeAsGain=on  AntiWindupMode=none  Kb=1  POutMin=[]  POutMax=[]  IOutMin=[]  IOutMax=[]  DOutMin=[]  DOutMax=[]  NOutMin=[]  NOutMax=[]  SumOutMin=[]  SumOutMax=[]  SaturationOutMin=[]  SaturationOutMax=[]  PParamMin=[]  PParamMax=[]  IParamMin=[]  IParamMax=[]  DParamMin=[]  DParamMax=[]  NParamMin=[]  NParamMax=[]  KbParamMin=[]  KbParamMax=[]  KtParamMin=[]  KtParamMax=[]  KbOutMin=[]  KbOutMax=[]  KtOutMin=[]  KtOutMax=[]  IntegratorOutMin=[]  IntegratorOutMax=[]  FilterOutMin=[]  FilterOutMax=[]  SumI1OutMin=[]  SumI1OutMax=[]  SumI2OutMin=[]  SumI2OutMax=[]  SumI3OutMin=[]  SumI3OutMax=[]  SumI4OutMin=[]  SumI4OutMax=[]  SumDOutMin=[]  SumDOutMax=[]  DifferentiatorOutMin=[]  DifferentiatorOutMax=[]  FilterDiffOutCoefMin=[]  FilterDiffOutCoefMax=[]  ReciprocalOutMin=[]  ReciprocalOutMax=[]  SumDenOutMin=[]  SumDenOutMax=[]  SumNumOutMin=[]  SumNumOutMax=[]  DivideOutMin=[]  DivideOutMax=[]  UdiffTsProdOutMin=[]  UdiffTsProdOutMax=[]  NTsProdOutMin=[]  NTsProdOutMax=[]  UintegralTsProdOutMin=[]  UintegralTsProdOutMax=[]  UngainTsProdOutMin=[]  UngainTsProdOutMax=[]  IntegratorContinuousStateAttributes=''  IntegratorStateMustResolveToSignalObject=off  IntegratorRTWStateStorageClass=Auto  FilterContinuousStateAttributes=''  FilterStateMustResolveToSignalObject=off  FilterRTWStateStorageClass=Auto  ParallelPVariant=InternalParameters  IdealPVariant=Disabled  IVariant=InternalParameters  DVariant=InternalParameters  IntegratorVariant=Discrete  SatVariant=Disabled  AWVariant=Passthrough  PCopyVariant=Disabled  TRVariant=Disabled  FdbkBlocksVariant=Forward  IdealPFdbkVariant=Disabled  SatFdbkVariant=Disabled  DerivativeFilterVariant=ForwardEulerFilter  NVariant=InternalParameters  NCopyVariant=Disabled  FilterICVariant=InternalICsFilter  IntegratorICVariant=InternalICs  ExternalResetVariant=Disabled  TRSumVariant=Passthrough  SumFdbkVariant=Disabled  SumVariant=Sum_PID  TsampFilterVariant=InternalTs  TsampNgainVariant=Passthrough  TsampIntegralVariant=Passthrough
  Saturation : Saturate  UpperLimit=1  LowerLimit=0
  Sum : Sum  Inputs=-+
  Tip-Speed Ratio MPPT : Subsystem
  LED_PWM : Outport
  WT_PWM : Outport  Port=2
  V_WT : Outport  Port=3
  wires:
  Sum/1 -> PID Controller/1  "d_lambda"
  Tip-Speed Ratio MPPT/5(d_turbine) -> Lambda calculation/5(d_turbine)
  r_LED/1 -> Gain/1
  Tip-Speed Ratio MPPT/3(V_w_data) -> Lambda calculation/3(V_w_data)
  Tip-Speed Ratio MPPT/2(omega) -> Lambda calculation/2(omega)
  r_WT/1 -> Lambda calculation/1(r_wind), Tip-Speed Ratio MPPT/1(r_wind)
  Constant/1 -> Sum/1
  Gain/1 -> LED_PWM/1
  Tip-Speed Ratio MPPT/1(V_WT) -> V_WT/1
  Lambda calculation/1(lambda) -> Sum/2
  Tip-Speed Ratio MPPT/4(r_wind_data) -> Lambda calculation/4(r_wind_data)
  Current/1 -> Tip-Speed Ratio MPPT/2(Current)
  Saturation/1 -> WT_PWM/1
  PID Controller/1 -> Saturation/1

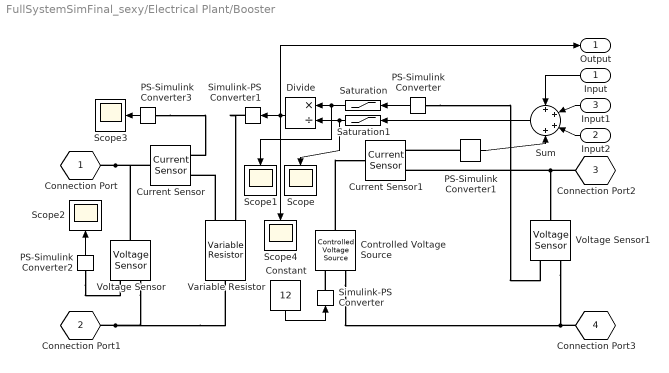
== system FullSystemSimFinal_sexy/Electrical Plant/Booster ==
  Input : Inport
  Input2 : Inport  Port=2
  Input1 : Inport  Port=3
  Constant : Constant  Value=12
  Controlled Voltage Source : fl_lib/Electrical/Electrical Sources/Controlled Voltage Source
  Current Sensor : fl_lib/Electrical/Electrical Sensors/Current Sensor
  Current Sensor1 : fl_lib/Electrical/Electrical Sensors/Current Sensor
  Divide : Product  Inputs=*/
  PS-Simulink Converter{,1..3} (4 alike) : nesl_utility/PS-Simulink Converter  PhysicalDomain=network_engine_domain  SubClassName=ps_output  LeftPortType=input  RightPortType=output  PseudoPeriodic=off  Frequencies=[]  Unit=inherit  AffineConversion=off
  Saturation : Saturate  UpperLimit=13  LowerLimit=0
  Saturation1 : Saturate  UpperLimit=2  LowerLimit=0.01
  Scope{,1..4} (5 alike) : Scope
  Simulink-PS Converter : nesl_utility/Simulink-PS Converter  PhysicalDomain=network_engine_domain  SubClassName=ps_input  LeftPortType=input  RightPortType=output  PseudoPeriodic=off  Frequencies=[]  NoiseDistribution=none  NoiseParameters=[]  Unit=1  AffineConversion=off  FilteringAndDerivatives=provide  SimscapeFilterOrder=1  InputFilterTimeConstant=0.001  UdotUserProvided=0
  Simulink-PS Converter1 : nesl_utility/Simulink-PS Converter  PhysicalDomain=network_engine_domain  SubClassName=ps_input  LeftPortType=input  RightPortType=output  PseudoPeriodic=off  Frequencies=[]  NoiseDistribution=none  NoiseParameters=[]  Unit=1  AffineConversion=off  FilteringAndDerivatives=filter  SimscapeFilterOrder=1  InputFilterTimeConstant=0.001  UdotUserProvided=0
  Sum : Sum  Inputs=++++
  Variable Resistor : fl_lib/Electrical/Electrical Elements/Variable Resistor  Rmin=0 Ohm  i_specify=off  i_priority=None  i=0 A  i_nominal_specify=off  i_nominal_unit=A  i_nominal_value=1  v_specify=off  v_priority=None  v=0 V  v_nominal_specify=off  v_nominal_unit=V  v_nominal_value=1
  Voltage Sensor : fl_lib/Electrical/Electrical Sensors/Voltage Sensor
  Voltage Sensor1 : fl_lib/Electrical/Electrical Sensors/Voltage Sensor
  Connection Port : PMIOPort  Tag=PMCPort  Side=Left
  Connection Port1 : PMIOPort  Tag=PMCPort  Port=2  Side=Left
  Connection Port2 : PMIOPort  Tag=PMCPort  Port=3  Side=Right
  Connection Port3 : PMIOPort  Tag=PMCPort  Port=4  Side=Right
  Output : Outport
  wires:
  Constant/1 -> Simulink-PS Converter/1
  PS-Simulink Converter2/1 -> Scope2/1
  PS-Simulink Converter3/1 -> Scope3/1
  Saturation/1 -> Scope1/1, Divide/1
  PS-Simulink Converter/1 -> Saturation/1
  Saturation1/1 -> Scope/1, Divide/2
  Divide/1 -> Output/1, Scope4/1, Simulink-PS Converter1/1
  Sum/1 -> Saturation1/1
  PS-Simulink Converter1/1 -> Sum/4
  Input/1 -> Sum/1
  Input1/1 -> Sum/2
  Input2/1 -> Sum/3
  connections:
  Voltage Sensor1/RConn2 -- Controlled Voltage Source/RConn2 -- Connection Port3/RConn1
  Connection Port1/RConn1 -- Voltage Sensor/RConn2 -- Variable Resistor/RConn1
  Connection Port/RConn1 -- Current Sensor/LConn1 -- Voltage Sensor/LConn1
  Simulink-PS Converter1/RConn1 -- Variable Resistor/LConn1
  Simulink-PS Converter/RConn1 -- Controlled Voltage Source/RConn1
  PS-Simulink Converter1/LConn1 -- Current Sensor1/RConn1
  Variable Resistor/LConn2 -- Current Sensor/RConn2
  PS-Simulink Converter/LConn1 -- Voltage Sensor1/RConn1
  PS-Simulink Converter2/LConn1 -- Voltage Sensor/RConn1
  PS-Simulink Converter3/LConn1 -- Current Sensor/RConn1
  Controlled Voltage Source/LConn1 -- Current Sensor1/LConn1
  Connection Port2/RConn1 -- Current Sensor1/RConn2 -- Voltage Sensor1/LConn1

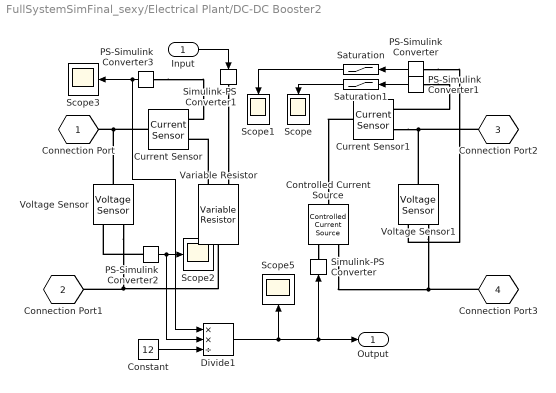
== system FullSystemSimFinal_sexy/Electrical Plant/DC-DC Booster2 ==
  Input : Inport
  Constant : Constant  Value=12
  Controlled Current Source : fl_lib/Electrical/Electrical Sources/Controlled Current Source
  Current Sensor : fl_lib/Electrical/Electrical Sensors/Current Sensor
  Current Sensor1 : fl_lib/Electrical/Electrical Sensors/Current Sensor
  Divide1 : Product  Inputs=**/
  PS-Simulink Converter{,1..3} (4 alike) : nesl_utility/PS-Simulink Converter  PhysicalDomain=network_engine_domain  SubClassName=ps_output  LeftPortType=input  RightPortType=output  PseudoPeriodic=off  Frequencies=[]  Unit=inherit  AffineConversion=off
  Saturation : Saturate  UpperLimit=13  LowerLimit=0
  Saturation1 : Saturate  UpperLimit=2  LowerLimit=0
  Scope{,1..3,5} (5 alike) : Scope
  Simulink-PS Converter : nesl_utility/Simulink-PS Converter  PhysicalDomain=network_engine_domain  SubClassName=ps_input  LeftPortType=input  RightPortType=output  PseudoPeriodic=off  Frequencies=[]  NoiseDistribution=none  NoiseParameters=[]  Unit=1  AffineConversion=off  FilteringAndDerivatives=filter  SimscapeFilterOrder=1  InputFilterTimeConstant=0.001  UdotUserProvided=0
  Simulink-PS Converter1 : nesl_utility/Simulink-PS Converter  PhysicalDomain=network_engine_domain  SubClassName=ps_input  LeftPortType=input  RightPortType=output  PseudoPeriodic=off  Frequencies=[]  NoiseDistribution=none  NoiseParameters=[]  Unit=1  AffineConversion=off  FilteringAndDerivatives=filter  SimscapeFilterOrder=1  InputFilterTimeConstant=0.001  UdotUserProvided=0
  Variable Resistor : fl_lib/Electrical/Electrical Elements/Variable Resistor  Rmin=0 Ohm  i_specify=off  i_priority=None  i=0 A  i_nominal_specify=off  i_nominal_unit=A  i_nominal_value=1  v_specify=off  v_priority=None  v=0 V  v_nominal_specify=off  v_nominal_unit=V  v_nominal_value=1
  Voltage Sensor : fl_lib/Electrical/Electrical Sensors/Voltage Sensor
  Voltage Sensor1 : fl_lib/Electrical/Electrical Sensors/Voltage Sensor
  Connection Port : PMIOPort  Tag=PMCPort  Side=Left
  Connection Port1 : PMIOPort  Tag=PMCPort  Port=2  Side=Left
  Connection Port2 : PMIOPort  Tag=PMCPort  Port=3  Side=Right
  Connection Port3 : PMIOPort  Tag=PMCPort  Port=4  Side=Right
  Output : Outport
  wires:
  Saturation/1 -> Scope1/1
  PS-Simulink Converter/1 -> Saturation/1
  PS-Simulink Converter1/1 -> Saturation1/1
  Saturation1/1 -> Scope/1
  Constant/1 -> Divide1/3
  PS-Simulink Converter2/1 -> Divide1/2, Scope2/1
  PS-Simulink Converter3/1 -> Scope3/1, Divide1/1
  Divide1/1 -> Output/1, Simulink-PS Converter/1, Scope5/1
  Input/1 -> Simulink-PS Converter1/1
  connections:
  Connection Port3/RConn1 -- Voltage Sensor1/RConn2 -- Controlled Current Source/RConn2
  Current Sensor1/RConn2 -- Connection Port2/RConn1 -- Voltage Sensor1/LConn1
  Voltage Sensor/RConn2 -- Variable Resistor/RConn1 -- Connection Port1/RConn1
  Current Sensor/LConn1 -- Voltage Sensor/LConn1 -- Connection Port/RConn1
  Simulink-PS Converter1/RConn1 -- Variable Resistor/LConn1
  Controlled Current Source/RConn1 -- Simulink-PS Converter/RConn1
  PS-Simulink Converter1/LConn1 -- Current Sensor1/RConn1
  Variable Resistor/LConn2 -- Current Sensor/RConn2
  PS-Simulink Converter/LConn1 -- Voltage Sensor1/RConn1
  PS-Simulink Converter2/LConn1 -- Voltage Sensor/RConn1
  PS-Simulink Converter3/LConn1 -- Current Sensor/RConn1
  Current Sensor1/LConn1 -- Controlled Current Source/LConn1

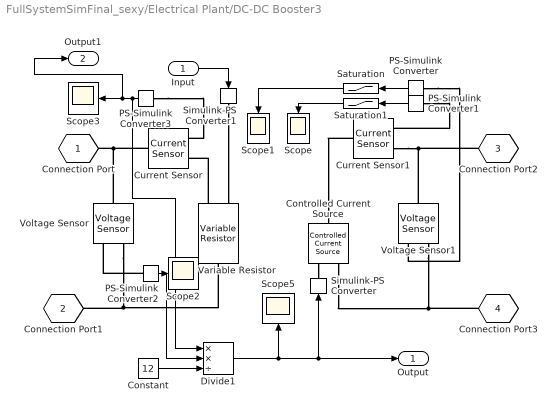
== system FullSystemSimFinal_sexy/Electrical Plant/DC-DC Booster3 ==
  Input : Inport
  Constant : Constant  Value=12
  Controlled Current Source : fl_lib/Electrical/Electrical Sources/Controlled Current Source
  Current Sensor : fl_lib/Electrical/Electrical Sensors/Current Sensor
  Current Sensor1 : fl_lib/Electrical/Electrical Sensors/Current Sensor
  Divide1 : Product  Inputs=**/
  PS-Simulink Converter{,1..3} (4 alike) : nesl_utility/PS-Simulink Converter  PhysicalDomain=network_engine_domain  SubClassName=ps_output  LeftPortType=input  RightPortType=output  PseudoPeriodic=off  Frequencies=[]  Unit=inherit  AffineConversion=off
  Saturation : Saturate  UpperLimit=13  LowerLimit=0
  Saturation1 : Saturate  UpperLimit=2  LowerLimit=0
  Scope{,1..3,5} (5 alike) : Scope
  Simulink-PS Converter : nesl_utility/Simulink-PS Converter  PhysicalDomain=network_engine_domain  SubClassName=ps_input  LeftPortType=input  RightPortType=output  PseudoPeriodic=off  Frequencies=[]  NoiseDistribution=none  NoiseParameters=[]  Unit=1  AffineConversion=off  FilteringAndDerivatives=filter  SimscapeFilterOrder=1  InputFilterTimeConstant=0.001  UdotUserProvided=0
  Simulink-PS Converter1 : nesl_utility/Simulink-PS Converter  PhysicalDomain=network_engine_domain  SubClassName=ps_input  LeftPortType=input  RightPortType=output  PseudoPeriodic=off  Frequencies=[]  NoiseDistribution=none  NoiseParameters=[]  Unit=1  AffineConversion=off  FilteringAndDerivatives=filter  SimscapeFilterOrder=1  InputFilterTimeConstant=0.001  UdotUserProvided=0
  Variable Resistor : fl_lib/Electrical/Electrical Elements/Variable Resistor  Rmin=0 Ohm  i_specify=off  i_priority=None  i=0 A  i_nominal_specify=off  i_nominal_unit=A  i_nominal_value=1  v_specify=off  v_priority=None  v=0 V  v_nominal_specify=off  v_nominal_unit=V  v_nominal_value=1
  Voltage Sensor : fl_lib/Electrical/Electrical Sensors/Voltage Sensor
  Voltage Sensor1 : fl_lib/Electrical/Electrical Sensors/Voltage Sensor
  Connection Port : PMIOPort  Tag=PMCPort  Side=Left
  Connection Port1 : PMIOPort  Tag=PMCPort  Port=2  Side=Left
  Connection Port2 : PMIOPort  Tag=PMCPort  Port=3  Side=Right
  Connection Port3 : PMIOPort  Tag=PMCPort  Port=4  Side=Right
  Output : Outport
  Output1 : Outport  Port=2
  wires:
  Saturation/1 -> Scope1/1
  PS-Simulink Converter/1 -> Saturation/1
  PS-Simulink Converter1/1 -> Saturation1/1
  Saturation1/1 -> Scope/1
  Constant/1 -> Divide1/3
  PS-Simulink Converter2/1 -> Divide1/2, Scope2/1
  PS-Simulink Converter3/1 -> Output1/1, Scope3/1, Divide1/1
  Input/1 -> Simulink-PS Converter1/1
  Divide1/1 -> Output/1, Simulink-PS Converter/1, Scope5/1
  connections:
  Connection Port3/RConn1 -- Voltage Sensor1/RConn2 -- Controlled Current Source/RConn2
  Current Sensor1/RConn2 -- Connection Port2/RConn1 -- Voltage Sensor1/LConn1
  Voltage Sensor/RConn2 -- Variable Resistor/RConn1 -- Connection Port1/RConn1
  Current Sensor/LConn1 -- Voltage Sensor/LConn1 -- Connection Port/RConn1
  Simulink-PS Converter1/RConn1 -- Variable Resistor/LConn1
  Controlled Current Source/RConn1 -- Simulink-PS Converter/RConn1
  PS-Simulink Converter1/LConn1 -- Current Sensor1/RConn1
  Variable Resistor/LConn2 -- Current Sensor/RConn2
  PS-Simulink Converter/LConn1 -- Voltage Sensor1/RConn1
  PS-Simulink Converter2/LConn1 -- Voltage Sensor/RConn1
  PS-Simulink Converter3/LConn1 -- Current Sensor/RConn1
  Current Sensor1/LConn1 -- Controlled Current Source/LConn1

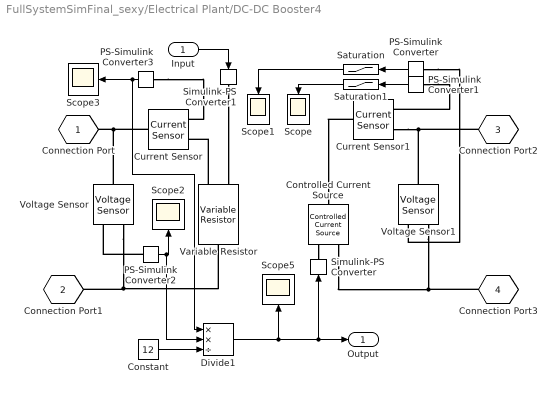
== system FullSystemSimFinal_sexy/Electrical Plant/DC-DC Booster4 ==
  Input : Inport
  Constant : Constant  Value=12
  Controlled Current Source : fl_lib/Electrical/Electrical Sources/Controlled Current Source
  Current Sensor : fl_lib/Electrical/Electrical Sensors/Current Sensor
  Current Sensor1 : fl_lib/Electrical/Electrical Sensors/Current Sensor
  Divide1 : Product  Inputs=**/
  PS-Simulink Converter{,1..3} (4 alike) : nesl_utility/PS-Simulink Converter  PhysicalDomain=network_engine_domain  SubClassName=ps_output  LeftPortType=input  RightPortType=output  PseudoPeriodic=off  Frequencies=[]  Unit=inherit  AffineConversion=off
  Saturation : Saturate  UpperLimit=13  LowerLimit=0
  Saturation1 : Saturate  UpperLimit=2  LowerLimit=0
  Scope{,1..3,5} (5 alike) : Scope
  Simulink-PS Converter : nesl_utility/Simulink-PS Converter  PhysicalDomain=network_engine_domain  SubClassName=ps_input  LeftPortType=input  RightPortType=output  PseudoPeriodic=off  Frequencies=[]  NoiseDistribution=none  NoiseParameters=[]  Unit=1  AffineConversion=off  FilteringAndDerivatives=filter  SimscapeFilterOrder=1  InputFilterTimeConstant=0.001  UdotUserProvided=0
  Simulink-PS Converter1 : nesl_utility/Simulink-PS Converter  PhysicalDomain=network_engine_domain  SubClassName=ps_input  LeftPortType=input  RightPortType=output  PseudoPeriodic=off  Frequencies=[]  NoiseDistribution=none  NoiseParameters=[]  Unit=1  AffineConversion=off  FilteringAndDerivatives=filter  SimscapeFilterOrder=1  InputFilterTimeConstant=0.001  UdotUserProvided=0
  Variable Resistor : fl_lib/Electrical/Electrical Elements/Variable Resistor  Rmin=0 Ohm  i_specify=off  i_priority=None  i=0 A  i_nominal_specify=off  i_nominal_unit=A  i_nominal_value=1  v_specify=off  v_priority=None  v=0 V  v_nominal_specify=off  v_nominal_unit=V  v_nominal_value=1
  Voltage Sensor : fl_lib/Electrical/Electrical Sensors/Voltage Sensor
  Voltage Sensor1 : fl_lib/Electrical/Electrical Sensors/Voltage Sensor
  Connection Port : PMIOPort  Tag=PMCPort  Side=Left
  Connection Port1 : PMIOPort  Tag=PMCPort  Port=2  Side=Left
  Connection Port2 : PMIOPort  Tag=PMCPort  Port=3  Side=Right
  Connection Port3 : PMIOPort  Tag=PMCPort  Port=4  Side=Right
  Output : Outport
  wires:
  Saturation/1 -> Scope1/1
  PS-Simulink Converter/1 -> Saturation/1
  PS-Simulink Converter1/1 -> Saturation1/1
  Saturation1/1 -> Scope/1
  Constant/1 -> Divide1/3
  PS-Simulink Converter2/1 -> Divide1/2, Scope2/1
  PS-Simulink Converter3/1 -> Scope3/1, Divide1/1
  Divide1/1 -> Simulink-PS Converter/1, Output/1, Scope5/1
  Input/1 -> Simulink-PS Converter1/1
  connections:
  Connection Port3/RConn1 -- Voltage Sensor1/RConn2 -- Controlled Current Source/RConn2
  Current Sensor1/RConn2 -- Connection Port2/RConn1 -- Voltage Sensor1/LConn1
  Voltage Sensor/RConn2 -- Variable Resistor/RConn1 -- Connection Port1/RConn1
  Current Sensor/LConn1 -- Voltage Sensor/LConn1 -- Connection Port/RConn1
  Simulink-PS Converter1/RConn1 -- Variable Resistor/LConn1
  Controlled Current Source/RConn1 -- Simulink-PS Converter/RConn1
  PS-Simulink Converter1/LConn1 -- Current Sensor1/RConn1
  Variable Resistor/LConn2 -- Current Sensor/RConn2
  PS-Simulink Converter/LConn1 -- Voltage Sensor1/RConn1
  PS-Simulink Converter2/LConn1 -- Voltage Sensor/RConn1
  PS-Simulink Converter3/LConn1 -- Current Sensor/RConn1
  Current Sensor1/LConn1 -- Controlled Current Source/LConn1

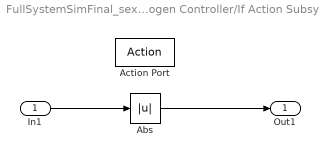
== system FullSystemSimFinal_sexy/Hydrogen Controller/If Action Subsystem ==
  In1 : Inport
  Action Port : ActionPort  ActionPortLabel=else
  Abs : Abs
  Out1 : Outport
  wires:
  In1/1 -> Abs/1
  Abs/1 -> Out1/1

== system FullSystemSimFinal_sexy/Hydrogen Controller/If Action Subsystem1 ==
  In1 : Inport
  Action Port : ActionPort  ActionPortLabel=if(u1 > 0)
  Out1 : Outport
  wires:
  In1/1 -> Out1/1

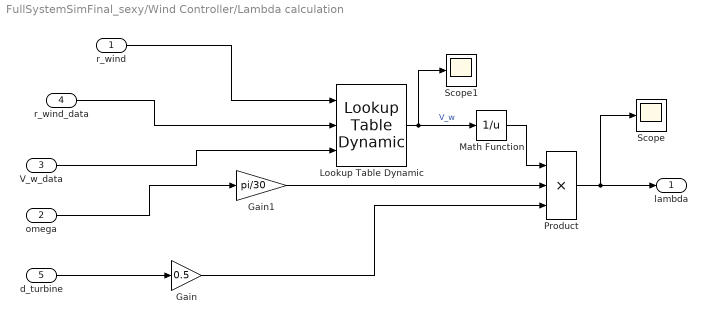
== system FullSystemSimFinal_sexy/Wind Controller/Lambda calculation ==
  r_wind : Inport
  omega : Inport  Port=2
  V_w_data : Inport  Port=3
  r_wind_data : Inport  Port=4
  d_turbine : Inport  Port=5
  Gain : Gain  Gain=0.5
  Gain1 : Gain  Gain=pi/30
  Lookup Table Dynamic : simulink/Lookup Tables/Lookup Table Dynamic  LookUpMeth=Interpolation-Use End Values  OutDataType=fixdt('double')  OutScaling=[]  OutputDataTypeScalingMode=Specify via dialog  OutDataTypeStr=double  DoSatur=off
  Math Function : Math  Operator=reciprocal  SignedPower=on  SaturateOnIntegerOverflow=on
  Product : Product  Inputs=3
  Scope : Scope
  Scope1 : Scope
  lambda : Outport
  wires:
  r_wind_data/1 -> Lookup Table Dynamic/2
  Product/1 -> Scope/1, lambda/1
  d_turbine/1 -> Gain/1
  V_w_data/1 -> Lookup Table Dynamic/3
  Math Function/1 -> Product/1
  r_wind/1 -> Lookup Table Dynamic/1
  omega/1 -> Gain1/1
  Lookup Table Dynamic/1 -> Scope1/1, Math Function/1  "V_w"
  Gain/1 -> Product/3
  Gain1/1 -> Product/2

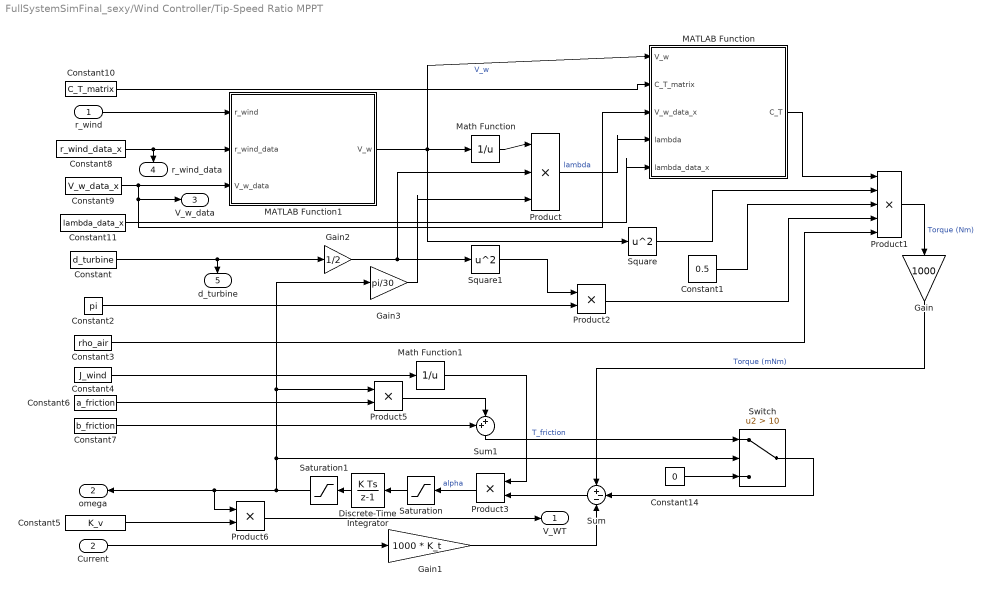
== system FullSystemSimFinal_sexy/Wind Controller/Tip-Speed Ratio MPPT ==
  r_wind : Inport
  Current : Inport  Port=2
  Constant : Constant  Value=d_turbine
  Constant1 : Constant  Value=0.5
  Constant10 : Constant  Value=C_T_matrix
  Constant11 : Constant  Value=lambda_data_x
  Constant14 : Constant  Value=0
  Constant2 : Constant  Value=pi
  Constant3 : Constant  Value=rho_air
  Constant4 : Constant  Value=J_wind  SampleTime=step_size
  Constant5 : Constant  Value=K_v
  Constant6 : Constant  Value=a_friction
  Constant7 : Constant  Value=b_friction  SampleTime=step_size
  Constant8 : Constant  Value=r_wind_data_x
  Constant9 : Constant  Value=V_w_data_x
  Discrete-Time Integrator : DiscreteIntegrator  InitialCondition=omega_0  SampleTime=-1  ICPrevOutput=DiscIntNeverNeededParam  ICPrevScaledInput=DiscIntNeverNeededParam
  Gain : Gain  Gain=1000
  Gain1 : Gain  Gain=1000 * K_t
  Gain2 : Gain  Gain=1/2
  Gain3 : Gain  Gain=pi/30
  MATLAB Function : MATLAB Function  TreatAsAtomicUnit=on
  MATLAB Function1 : MATLAB Function  TreatAsAtomicUnit=on
  Math Function : Math  Operator=reciprocal  SignedPower=on  SaturateOnIntegerOverflow=on
  Math Function1 : Math  Operator=reciprocal  SignedPower=on  SaturateOnIntegerOverflow=on
  Product : Product  Inputs=3
  Product1 : Product  Inputs=5
  Product{2..3,5..6} (4 alike) : Product
  Saturation : Saturate  UpperLimit=10000  LowerLimit=-10000
  Saturation1 : Saturate  UpperLimit=3000  LowerLimit=1000
  Square : Math  Operator=square  SignedPower=on  SaturateOnIntegerOverflow=on
  Square1 : Math  Operator=square  SignedPower=on  SaturateOnIntegerOverflow=on
  Sum : Sum  Inputs=+--
  Sum1 : Sum  Inputs=++|
  Switch : Switch  Criteria=u2 > Threshold  Threshold=10
  V_WT : Outport
  omega : Outport  Port=2
  V_w_data : Outport  Port=3
  r_wind_data : Outport  Port=4
  d_turbine : Outport  Port=5
  wires:
  Switch/1 -> Sum/2
  Gain1/1 -> Sum/3
  Product3/1 -> Saturation/1  "alpha"
  Math Function/1 -> Product/1
  Constant10/1 -> MATLAB Function/2(C_T_matrix)
  Product2/1 -> Product1/4
  Constant5/1 -> Product6/2
  Math Function1/1 -> Product3/1
  Constant6/1 -> Product5/2
  Sum/1 -> Product3/2
  Constant2/1 -> Product2/2
  Current/1 -> Gain1/1
  Constant4/1 -> Math Function1/1
  Square/1 -> Product1/2
  Constant3/1 -> Product1/5
  Constant7/1 -> Sum1/1
  r_wind/1 -> MATLAB Function1/1(r_wind)
  Product/1 -> MATLAB Function/4(lambda)  "lambda"
  Constant/1 -> Gain2/1, d_turbine/1
  Constant8/1 -> MATLAB Function1/2(r_wind_data), r_wind_data/1
  Constant9/1 -> V_w_data/1, MATLAB Function/3(V_w_data_x), MATLAB Function1/3(V_w_data)
  Product6/1 -> V_WT/1
  Square1/1 -> Product2/1
  MATLAB Function/1(C_T) -> Product1/1
  Gain/1 -> Sum/1  "Torque (mNm)"
  Product5/1 -> Sum1/2
  Constant11/1 -> MATLAB Function/5(lambda_data_x)
  Constant14/1 -> Switch/3
  Saturation/1 -> Discrete-Time Integrator/1
  Constant1/1 -> Product1/3
  Sum1/1 -> Switch/1  "T_friction"
  Product1/1 -> Gain/1  "Torque (Nm)"
  MATLAB Function1/1(V_w) -> Math Function/1, MATLAB Function/1(V_w), Square/1  "V_w"
  Gain2/1 -> Square1/1, Product/2
  Gain3/1 -> Product/3
  Saturation1/1 -> Switch/2, Gain3/1, Product5/1, Product6/1, omega/1
  Discrete-Time Integrator/1 -> Saturation1/1

== matlab function FullSystemSimFinal_sexy/Wind Controller/Tip-Speed Ratio MPPT/MATLAB Function1 ==
  data: r_wind input; V_w output; r_wind_data input; V_w_data input
function V_w = TableLookup(r_wind,r_wind_data,V_w_data)

V_w = interp1(r_wind_data,V_w_data,min(r_wind,0.999999));

== matlab function FullSystemSimFinal_sexy/Wind Controller/Tip-Speed Ratio MPPT/MATLAB Function ==
  data: V_w input; C_T output; C_T_matrix input; V_w_data_x input; lambda input; lambda_data_x input
function C_T = MatrixLookUp(V_w,C_T_matrix,V_w_data_x,lambda,lambda_data_x)

lambda = min( max(lambda, 0), 10);

C_T = interp1(lambda_data_x,interp1(V_w_data_x,C_T_matrix,V_w),lambda);

== matlab function FullSystemSimFinal_sexy/Solar Controller/MATLAB Function ==
  data: r_SP input; I_SP output; R_load input; r_solar_data input; V_oc_data input; I_sc_data input; V_mp_data input; I_mp_data input; R_mp_data input
function I_SP = SolarInterp(r_SP,R_load, r_solar_data, V_oc_data, I_sc_data, V_mp_data, I_mp_data, R_mp_data)
V_oc = interp1(r_solar_data,V_oc_data,r_SP);
I_sc = interp1(r_solar_data,I_sc_data,r_SP);
V_mp = interp1(r_solar_data,V_mp_data,r_SP);
I_mp = interp1(r_solar_data,I_mp_data,r_SP);
R_mp = interp1(r_solar_data,R_mp_data,r_SP);

if (R_load < R_mp )
    I_SP = max(I_sc/((1/R_load)+((I_sc-I_mp)/V_mp)) / R_load, 0);
else
    I_SP = max((I_mp+I_mp*V_mp/(V_oc-V_mp))/((1/R_load)+I_mp/(V_oc-V_mp)) / R_load, 0);
end
